simulink model "SST_FINAL_SIMULINK"  (R2017b)
settings: Solver=ode14x  StartTime=0.0  StopTime=120/60  MaxStep=1e-4  RelTol=1e-3
values from neighbouring files (symbols this model uses):
  C_3P4L = (Potencia_nominal)/(2*pi*60*0.1*((Entrada)^2))    (= 0.00858724363662)    [SST_FINAL.m]
  C_HB = 50000/(0.6*60*pi*(11397^2))    (= 3.40358447746e-06)    [SST_FINAL.m]
  ca = 1/(L*a)    [SST_FINAL.m]
  CDAB1 = 50*(Pnom/3)/(Vmin_DAB1^2*Fsw_DAB)    [SST_FINAL.m]
  CDAB2 = 50*(Pnom/3)/(Vmin_DAB2^2*Fsw_DAB)    [SST_FINAL.m]
  E = Nm*Vout_HB    (= 11397)    [SST_FINAL.m]
  Fsw_DAB = 30e3    (= 30000)    [SST_FINAL.m]
  Fsw_HB = 15e3    (= 15000)    [SST_FINAL.m]
  Fsw_NPC = 5040    [SST_FINAL.m]
  Inom_HB = (50e3/(13200*sqrt(3)))*sqrt(2)    [SST_FINAL.m]
  Kc_I = H_infI    [SST_FINAL.m]
  Kc_V = H_infV    [SST_FINAL.m]
  KcI_DAB = H_infI_DAB    [SST_FINAL.m]
  KcV_DAB = H_infV_DAB    [SST_FINAL.m]
  Ki = 2.5641    [SST_FINAL.m]
  Kp = 0.00138    [SST_FINAL.m]
  L = ((0.03*Entrada))/((2*pi*60)*(Imax))    [SST_FINAL.m]
  L_DAB = (1/Ntr)*VDAB1*VDAB2*D*(1-D)/(2*Fsw_DAB*(Pnom/3))    (= 2.89591875e-05)    [SST_FINAL.m]
  L_HB = 50e-3    (= 0.05)    [SST_FINAL.m]
  m = (2*Voltaje_pico)/Entrada    [SST_FINAL.m]
  Pnom = 50e3    (= 50000)    [SST_FINAL.m]
  R_DAB = 30e3*2*pi*L_DAB*0.1    (= 0.545867824224)    [SST_FINAL.m]
  R_HB = 120*pi*L_HB*0.05    (= 0.942477796077)    [SST_FINAL.m]
  R_LOAD2 = VDAB2^2/(Pnom/3)    (= 9.26694)    [SST_FINAL.m]
  tauI_I = 1/(2*pi*F_lagI)    (= 0.00265258238486)    [SST_FINAL.m]
  tauI_V = 1/(2*pi*F_LagV)    (= 0.00039788735773)    [SST_FINAL.m]
  tauII_DAB = 1/(2*pi*F_lagI_DAB)    (= 0.00265258238486)    [SST_FINAL.m]
  tauIV_DAB = 1/(2*pi*F_lagV_DAB)    (= 0.265258238486)    [SST_FINAL.m]
  Ts = 1/(200*Fsw_DAB)    (= 1.66666666667e-07)    [SST_FINAL.m]
  uLmt_dDAB = 0.5    [SST_FINAL.m]
  uLmt_I = 0.05    [SST_FINAL.m]
  uLmt_V = Inom_HB    [SST_FINAL.m]
  VDAB1 = 11397    [SST_FINAL.m]
  VDAB2 = 393    [SST_FINAL.m]
  Vp = Entrada/2    (= 196.5)    [SST_FINAL.m]
  W = 120*pi    (= 376.991118431)    [SST_FINAL.m]
  w = 120*pi    (= 376.991118431)    [SST_FINAL.m]
libraries: powerlib x102, powerlib_meascontrol x26, simulink x16, dspstat3 x3
(part 2 of 2)

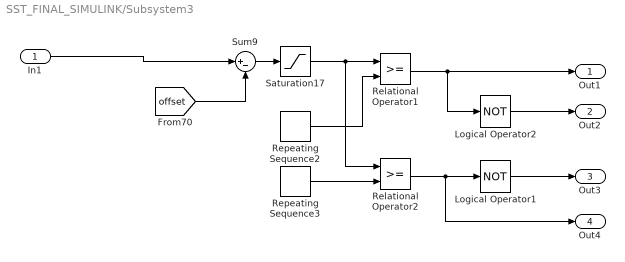
== system SST_FINAL_SIMULINK/Subsystem3 ==
  In1 : Inport
  Logical Operator1 : Logic  Operator=NOT  AllPortsSameDT=off  OutDataTypeStr=boolean
  Logical Operator2 : Logic  Operator=NOT  AllPortsSameDT=off  OutDataTypeStr=boolean
  Relational Operator1 : RelationalOperator  ZeroCross=off  RndMeth=Nearest
  Relational Operator2 : RelationalOperator  ZeroCross=off  RndMeth=Nearest
  Repeating Sequence2 : simulink/Sources/Repeating Sequence  rep_seq_t=[0 0.5/Fsw_NPC 1/Fsw_NPC]  rep_seq_y=[ 0 1 0 ]
  Repeating Sequence3 : simulink/Sources/Repeating Sequence  rep_seq_t=[0 0.5/Fsw_NPC 1/Fsw_NPC]  rep_seq_y=[-1 0 -1]
  Saturation17 : Saturate  UpperLimit=m  LowerLimit=-m  ZeroCross=off
  Sum9 : Sum  Inputs=|+-
  Out1 : Outport
  Out2 : Outport  Port=2
  Out3 : Outport  Port=3
  Out4 : Outport  Port=4
  wires:
  Saturation17/1 -> Relational Operator2/1, Relational Operator1/1
  Relational Operator1/1 -> Out1/1, Logical Operator2/1
  Repeating Sequence2/1 -> Relational Operator1/2
  Sum9/1 -> Saturation17/1
  Logical Operator2/1 -> Out2/1
  Logical Operator1/1 -> Out3/1
  [offset] -> Sum9/2
  Relational Operator2/1 -> Out4/1, Logical Operator1/1
  In1/1 -> Sum9/1
  Repeating Sequence3/1 -> Relational Operator2/2

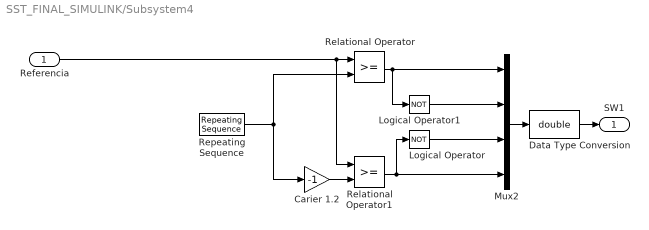
== system SST_FINAL_SIMULINK/Subsystem4 ==
  Referencia : Inport
  Carier 1.2 : Gain  Gain=-1
  Data Type Conversion : DataTypeConversion  OutDataTypeStr=double
  Logical Operator : Logic  Operator=NOT  IconShape=distinctive  AllPortsSameDT=off  OutDataTypeStr=boolean
  Logical Operator1 : Logic  Operator=NOT  IconShape=distinctive  AllPortsSameDT=off  OutDataTypeStr=boolean
  Mux2 : Mux
  Relational Operator : RelationalOperator  OutDataTypeStr=boolean  RndMeth=Simplest
  Relational Operator1 : RelationalOperator  OutDataTypeStr=boolean  RndMeth=Simplest
  Repeating Sequence : simulink/Sources/Repeating Sequence  rep_seq_t=[0 0.5 1]/Fsw_HB  rep_seq_y=[0 1 0]
  SW1 : Outport
  wires:
  Referencia/1 -> Relational Operator/1, Relational Operator1/1
  Repeating Sequence/1 -> Carier 1.2/1, Relational Operator/2
  Logical Operator1/1 -> Mux2/2
  Data Type Conversion/1 -> SW1/1
  Mux2/1 -> Data Type Conversion/1
  Logical Operator/1 -> Mux2/3
  Relational Operator/1 -> Mux2/1, Logical Operator1/1
  Carier 1.2/1 -> Relational Operator1/2
  Relational Operator1/1 -> Mux2/4, Logical Operator/1

== system SST_FINAL_SIMULINK/Subsystem5 ==
  In1 : Inport
  In2 : Inport  Port=2
  IGBT3 : powerlib/Power Electronics/IGBT  Ron=0.000000001  Lon=0  Vf=0  Tf=1e-6  Tt=2e-6  IC=0  Rs=inf  Cs=inf  Measurements=off
  IGBT4 : powerlib/Power Electronics/IGBT  Ron=0.000000001  Lon=0  Vf=0  Tf=1e-6  Tt=2e-6  IC=0  Rs=1e5  Cs=inf  Measurements=off
  Conn1 : PMIOPort  Port=1  Side=Left
  Conn2 : PMIOPort  Port=2  Side=Right
  Conn3 : PMIOPort  Port=3  Side=Left
  wires:
  In1/1 -> IGBT3/1
  In2/1 -> IGBT4/1
  connections:
  Conn3/RConn1 -- IGBT4/LConn1 -- IGBT3/RConn1
  IGBT4/RConn1 -- Conn2/RConn1
  IGBT3/LConn1 -- Conn1/RConn1

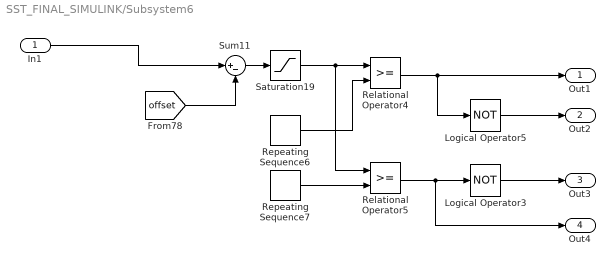
== system SST_FINAL_SIMULINK/Subsystem6 ==
  In1 : Inport
  Logical Operator3 : Logic  Operator=NOT  AllPortsSameDT=off  OutDataTypeStr=boolean
  Logical Operator5 : Logic  Operator=NOT  AllPortsSameDT=off  OutDataTypeStr=boolean
  Relational Operator4 : RelationalOperator  ZeroCross=off  RndMeth=Nearest
  Relational Operator5 : RelationalOperator  ZeroCross=off  RndMeth=Nearest
  Repeating Sequence6 : simulink/Sources/Repeating Sequence  rep_seq_t=[0 0.5/Fsw_NPC 1/Fsw_NPC]  rep_seq_y=[ 0 1 0 ]
  Repeating Sequence7 : simulink/Sources/Repeating Sequence  rep_seq_t=[0 0.5/Fsw_NPC 1/Fsw_NPC]  rep_seq_y=[-1 0 -1]
  Saturation19 : Saturate  UpperLimit=m  LowerLimit=-m  ZeroCross=off
  Sum11 : Sum  Inputs=|+-
  Out1 : Outport
  Out2 : Outport  Port=2
  Out3 : Outport  Port=3
  Out4 : Outport  Port=4
  wires:
  Sum11/1 -> Saturation19/1
  Relational Operator5/1 -> Out4/1, Logical Operator3/1
  Logical Operator3/1 -> Out3/1
  Saturation19/1 -> Relational Operator5/1, Relational Operator4/1
  In1/1 -> Sum11/1
  [offset] -> Sum11/2
  Repeating Sequence6/1 -> Relational Operator4/2
  Repeating Sequence7/1 -> Relational Operator5/2
  Relational Operator4/1 -> Out1/1, Logical Operator5/1
  Logical Operator5/1 -> Out2/1

== system SST_FINAL_SIMULINK/Subsystem7 ==
  In1 : Inport
  In2 : Inport  Port=2
  IGBT1 : powerlib/Power Electronics/IGBT  Ron=0.000000001  Lon=0  Vf=0  Tf=1e-6  Tt=2e-6  IC=0  Rs=1e5  Cs=inf  Measurements=off
  IGBT3 : powerlib/Power Electronics/IGBT  Ron=0.000000001  Lon=0  Vf=0  Tf=1e-6  Tt=2e-6  IC=0  Rs=inf  Cs=inf  Measurements=off
  Conn1 : PMIOPort  Port=1  Side=Left
  Conn2 : PMIOPort  Port=2  Side=Right
  Conn3 : PMIOPort  Port=3  Side=Left
  wires:
  In1/1 -> IGBT3/1
  In2/1 -> IGBT1/1
  connections:
  Conn3/RConn1 -- IGBT3/RConn1 -- IGBT1/LConn1
  IGBT1/RConn1 -- Conn2/RConn1
  IGBT3/LConn1 -- Conn1/RConn1

== system SST_FINAL_SIMULINK/Subsystem8 ==
  In1 : Inport
  In2 : Inport  Port=2
  IGBT3 : powerlib/Power Electronics/IGBT  Ron=0.000000001  Lon=0  Vf=0  Tf=1e-6  Tt=2e-6  IC=0  Rs=1e5  Cs=inf  Measurements=off
  IGBT4 : powerlib/Power Electronics/IGBT  Ron=0.000000001  Lon=0  Vf=0  Tf=1e-6  Tt=2e-6  IC=0  Rs=inf  Cs=inf  Measurements=off
  Conn1 : PMIOPort  Port=1  Side=Left
  Conn2 : PMIOPort  Port=2  Side=Right
  Conn3 : PMIOPort  Port=3  Side=Left
  wires:
  In2/1 -> IGBT3/1
  In1/1 -> IGBT4/1
  connections:
  IGBT4/LConn1 -- Conn1/RConn1
  IGBT3/RConn1 -- Conn2/RConn1
  Conn3/RConn1 -- IGBT3/LConn1 -- IGBT4/RConn1

== system SST_FINAL_SIMULINK/Subsystem9 ==
  In1 : Inport
  In2 : Inport  Port=2
  IGBT3 : powerlib/Power Electronics/IGBT  Ron=0.000000001  Lon=0  Vf=0  Tf=1e-6  Tt=2e-6  IC=0  Rs=inf  Cs=inf  Measurements=off
  IGBT4 : powerlib/Power Electronics/IGBT  Ron=0.000000001  Lon=0  Vf=0  Tf=1e-6  Tt=2e-6  IC=0  Rs=1e5  Cs=inf  Measurements=off
  Conn1 : PMIOPort  Port=1  Side=Left
  Conn2 : PMIOPort  Port=2  Side=Right
  Conn3 : PMIOPort  Port=3  Side=Left
  wires:
  In2/1 -> IGBT4/1
  In1/1 -> IGBT3/1
  connections:
  IGBT3/LConn1 -- Conn1/RConn1
  IGBT4/RConn1 -- Conn2/RConn1
  Conn3/RConn1 -- IGBT4/LConn1 -- IGBT3/RConn1

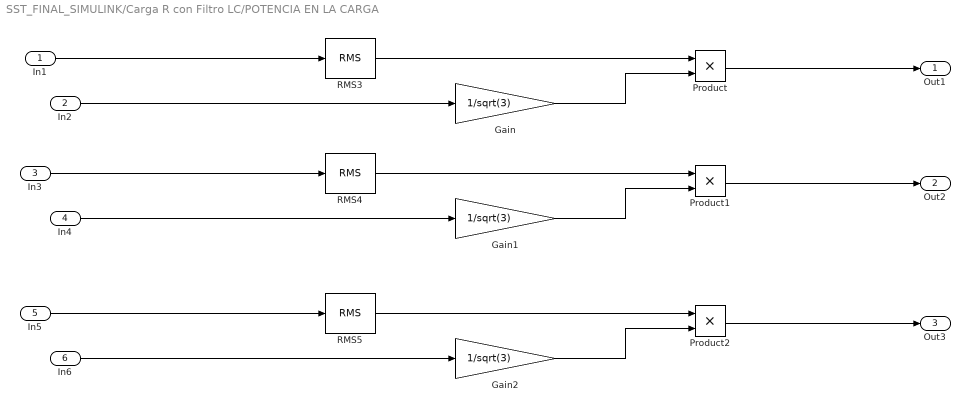
== system SST_FINAL_SIMULINK/Carga R con Filtro LC/POTENCIA EN LA CARGA  ==
  In1 : Inport
  In2 : Inport  Port=2
  In3 : Inport  Port=3
  In4 : Inport  Port=4
  In5 : Inport  Port=5
  In6 : Inport  Port=6
  Gain : Gain  Gain=1/sqrt(3)
  Gain1 : Gain  Gain=1/sqrt(3)
  Gain2 : Gain  Gain=1/sqrt(3)
  Product : Product
  Product1 : Product
  Product2 : Product
  RMS3 : powerlib_meascontrol/Measurements/RMS  TrueRMS=off  Freq=60  RMSInit=0  Ts=0
  RMS4 : powerlib_meascontrol/Measurements/RMS  TrueRMS=off  Freq=60  RMSInit=0  Ts=0
  RMS5 : powerlib_meascontrol/Measurements/RMS  TrueRMS=off  Freq=60  RMSInit=0  Ts=0
  Out1 : Outport
  Out2 : Outport  Port=2
  Out3 : Outport  Port=3
  wires:
  Gain1/1 -> Product1/2
  In4/1 -> Gain1/1
  In6/1 -> Gain2/1
  Product2/1 -> Out3/1
  Gain/1 -> Product/2
  RMS4/1 -> Product1/1
  RMS5/1 -> Product2/1
  Product/1 -> Out1/1
  RMS3/1 -> Product/1
  In3/1 -> RMS4/1
  In1/1 -> RMS3/1
  Product1/1 -> Out2/1
  Gain2/1 -> Product2/2
  In2/1 -> Gain/1
  In5/1 -> RMS5/1

== matlab function SST_FINAL_SIMULINK/CONTROL_ID_buck2 ==
  settings: updateMethod=DISCRETE  sampleTime=Ts
  data: yCur input; uCur output; rCur input; KcV_DAB parameter; tauIV_DAB parameter; Ts parameter
function uCur= PIV(yCur,rCur,KcV_DAB,tauIV_DAB,Ts)

persistent uPast yPast rPast
if isempty(uPast),uPast=0;end
if isempty(yPast),yPast=0;end
if isempty(rPast),rPast=0;end

% uCur=uPast+Kc_v*((rCur-yCur)-(rPast-yPast))+(Kc_v*Ts/tauI_v)*(rCur-yCur)+Kd_v*((rCur-yCur)-(rPast-yPast))/Ts;
uCur=uPast+KcV_DAB*((rCur-yCur)-(rPast-yPast))+(KcV_DAB*Ts/tauIV_DAB)*(rCur-yCur);

uPast=uCur;
yPast=yCur;
rPast=rCur;

== matlab function SST_FINAL_SIMULINK/MATLAB Function5 ==
  settings: updateMethod=DISCRETE  sampleTime=Ts
  data: yCur input; uCur output; rCur input; Kc_I parameter; tauI_I parameter; Ts parameter; uLmt_I parameter
function uCur= PIV(yCur,rCur,Kc_I,tauI_I,Ts,uLmt_I)

persistent uPast yPast rPast
if isempty(uPast),uPast=0;end
if isempty(yPast),yPast=0;end
if isempty(rPast),rPast=0;end

uCur=uPast+Kc_I*((rCur-yCur)-(rPast-yPast))+(Kc_I*Ts/tauI_I)*(rCur-yCur);

if (uCur>uLmt_I)
uCur=uLmt_I;
end
if (uCur<-uLmt_I)
uCur= -uLmt_I;
end

uPast=uCur;
yPast=yCur;
rPast=rCur;

== matlab function SST_FINAL_SIMULINK/CONTROL_ID_buck3 ==
  settings: updateMethod=DISCRETE  sampleTime=Ts
  data: yCur input; uCur output; rCur input; KcV_DAB parameter; tauIV_DAB parameter; Ts parameter
function uCur= PIV(yCur,rCur,KcV_DAB,tauIV_DAB,Ts)

persistent uPast yPast rPast
if isempty(uPast),uPast=0;end
if isempty(yPast),yPast=0;end
if isempty(rPast),rPast=0;end

% uCur=uPast+Kc_v*((rCur-yCur)-(rPast-yPast))+(Kc_v*Ts/tauI_v)*(rCur-yCur)+Kd_v*((rCur-yCur)-(rPast-yPast))/Ts;
uCur=uPast+KcV_DAB*((rCur-yCur)-(rPast-yPast))+(KcV_DAB*Ts/tauIV_DAB)*(rCur-yCur);

uPast=uCur;
yPast=yCur;
rPast=rCur;

== matlab function SST_FINAL_SIMULINK/CONTROL_ID_buck5 ==
  settings: updateMethod=DISCRETE  sampleTime=Ts
  data: yCur input; uCur output; rCur input; KcI_DAB parameter; tauII_DAB parameter; Ts parameter; uLmt_dDAB parameter
function uCur= PIV(yCur,rCur,KcI_DAB,tauII_DAB,Ts,uLmt_dDAB)

persistent uPast yPast rPast
if isempty(uPast),uPast=0;end
if isempty(yPast),yPast=0;end
if isempty(rPast),rPast=0;end

% uCur=uPast+Kc_v*((rCur-yCur)-(rPast-yPast))+(Kc_v*Ts/tauI_v)*(rCur-yCur)+Kd_v*((rCur-yCur)-(rPast-yPast))/Ts;
uCur=uPast+KcI_DAB*((rCur-yCur)-(rPast-yPast))+(KcI_DAB*Ts/tauII_DAB)*(rCur-yCur);

if (uCur>uLmt_dDAB)
uCur=uLmt_dDAB;
end
if (uCur<-uLmt_dDAB)
uCur= -uLmt_dDAB;
end

uPast=uCur;
yPast=yCur;
rPast=rCur;

== matlab function SST_FINAL_SIMULINK/MATLAB Function2 ==
  settings: updateMethod=DISCRETE  sampleTime=Ts
  data: Carrier_dab input; S_dab output; d_dab input
function S_dab = fcn(Carrier_dab,d_dab)


    
if Carrier_dab>=0 && Carrier_dab<pi
    if d_dab>Carrier_dab
        S_dab=[1 0 0 1 0 1 1 0];
    else
        S_dab=[1 0 0 1 1 0 0 1];
    end
else
    if (d_dab+pi)>Carrier_dab
        S_dab=[0 1 1 0 1 0 0 1];
    else
        S_dab=[0 1 1 0 0 1 1 0];
    end
end

end

== matlab function SST_FINAL_SIMULINK/MATLAB Function3 ==
  settings: updateMethod=DISCRETE  sampleTime=Ts
  data: Carrier_dab input; S_dab output; d_dab input
function S_dab = fcn(Carrier_dab,d_dab)


    
if Carrier_dab>=0 && Carrier_dab<pi
    if d_dab>Carrier_dab
        S_dab=[1 0 0 1 0 1 1 0];
    else
        S_dab=[1 0 0 1 1 0 0 1];
    end
else
    if (d_dab+pi)>Carrier_dab
        S_dab=[0 1 1 0 1 0 0 1];
    else
        S_dab=[0 1 1 0 0 1 1 0];
    end
end

end

== matlab function SST_FINAL_SIMULINK/MATLAB Function6 ==
  settings: updateMethod=DISCRETE  sampleTime=Ts
  data: yCur input; uCur output; rCur input; Kc_I parameter; tauI_I parameter; Ts parameter; uLmt_I parameter
function uCur= PIV(yCur,rCur,Kc_I,tauI_I,Ts,uLmt_I)

persistent uPast yPast rPast
if isempty(uPast),uPast=0;end
if isempty(yPast),yPast=0;end
if isempty(rPast),rPast=0;end

uCur=uPast+Kc_I*((rCur-yCur)-(rPast-yPast))+(Kc_I*Ts/tauI_I)*(rCur-yCur);

if (uCur>uLmt_I)
uCur=uLmt_I;
end
if (uCur<-uLmt_I)
uCur= -uLmt_I;
end

uPast=uCur;
yPast=yCur;
rPast=rCur;

== matlab function SST_FINAL_SIMULINK/CONTROL_ID_buck6 ==
  settings: updateMethod=DISCRETE  sampleTime=Ts
  data: yCur input; uCur output; rCur input; KcI_DAB parameter; tauII_DAB parameter; Ts parameter; uLmt_dDAB parameter
function uCur= PIV(yCur,rCur,KcI_DAB,tauII_DAB,Ts,uLmt_dDAB)

persistent uPast yPast rPast
if isempty(uPast),uPast=0;end
if isempty(yPast),yPast=0;end
if isempty(rPast),rPast=0;end

% uCur=uPast+Kc_v*((rCur-yCur)-(rPast-yPast))+(Kc_v*Ts/tauI_v)*(rCur-yCur)+Kd_v*((rCur-yCur)-(rPast-yPast))/Ts;
uCur=uPast+KcI_DAB*((rCur-yCur)-(rPast-yPast))+(KcI_DAB*Ts/tauII_DAB)*(rCur-yCur);

if (uCur>uLmt_dDAB)
uCur=uLmt_dDAB;
end
if (uCur<-uLmt_dDAB)
uCur= -uLmt_dDAB;
end

uPast=uCur;
yPast=yCur;
rPast=rCur;

== matlab function SST_FINAL_SIMULINK/MATLAB Function4 ==
  settings: updateMethod=DISCRETE  sampleTime=Ts
  data: Carrier_dab input; S_dab output; d_dab input
function S_dab = fcn(Carrier_dab,d_dab)


    
if Carrier_dab>=0 && Carrier_dab<pi
    if d_dab>Carrier_dab
        S_dab=[1 0 0 1 0 1 1 0];
    else
        S_dab=[1 0 0 1 1 0 0 1];
    end
else
    if (d_dab+pi)>Carrier_dab
        S_dab=[0 1 1 0 1 0 0 1];
    else
        S_dab=[0 1 1 0 0 1 1 0];
    end
end

end

== matlab function SST_FINAL_SIMULINK/MATLAB Function7 ==
  settings: updateMethod=DISCRETE  sampleTime=Ts
  data: yCur input; uCur output; rCur input; Kc_V parameter; tauI_V parameter; Ts parameter; uLmt_V parameter
function uCur= PIV(yCur,rCur,Kc_V,tauI_V,Ts,uLmt_V)

persistent uPast yPast rPast
if isempty(uPast),uPast=0;end
if isempty(yPast),yPast=0;end
if isempty(rPast),rPast=0;end

uCur=uPast+Kc_V*((rCur-yCur)-(rPast-yPast))+(Kc_V*Ts/tauI_V)*(rCur-yCur);

if (uCur>uLmt_V)
uCur=uLmt_V;
end
if (uCur<-uLmt_V)
uCur= -uLmt_V;
end

uPast=uCur;
yPast=yCur;
rPast=rCur;

== matlab function SST_FINAL_SIMULINK/CONTROL_ID_buck8 ==
  settings: updateMethod=DISCRETE  sampleTime=Ts
  data: yCur input; uCur output; rCur input; KcI_DAB parameter; tauII_DAB parameter; Ts parameter; uLmt_dDAB parameter
function uCur= PIV(yCur,rCur,KcI_DAB,tauII_DAB,Ts,uLmt_dDAB)

persistent uPast yPast rPast
if isempty(uPast),uPast=0;end
if isempty(yPast),yPast=0;end
if isempty(rPast),rPast=0;end

% uCur=uPast+Kc_v*((rCur-yCur)-(rPast-yPast))+(Kc_v*Ts/tauI_v)*(rCur-yCur)+Kd_v*((rCur-yCur)-(rPast-yPast))/Ts;
uCur=uPast+KcI_DAB*((rCur-yCur)-(rPast-yPast))+(KcI_DAB*Ts/tauII_DAB)*(rCur-yCur);

if (uCur>uLmt_dDAB)
uCur=uLmt_dDAB;
end
if (uCur<-uLmt_dDAB)
uCur= -uLmt_dDAB;
end

uPast=uCur;
yPast=yCur;
rPast=rCur;

== matlab function SST_FINAL_SIMULINK/CONTROL_ID_buck9 ==
  settings: updateMethod=DISCRETE  sampleTime=Ts
  data: yCur input; uCur output; rCur input; KcV_DAB parameter; tauIV_DAB parameter; Ts parameter
function uCur= PIV(yCur,rCur,KcV_DAB,tauIV_DAB,Ts)

persistent uPast yPast rPast
if isempty(uPast),uPast=0;end
if isempty(yPast),yPast=0;end
if isempty(rPast),rPast=0;end

% uCur=uPast+Kc_v*((rCur-yCur)-(rPast-yPast))+(Kc_v*Ts/tauI_v)*(rCur-yCur)+Kd_v*((rCur-yCur)-(rPast-yPast))/Ts;
uCur=uPast+KcV_DAB*((rCur-yCur)-(rPast-yPast))+(KcV_DAB*Ts/tauIV_DAB)*(rCur-yCur);

uPast=uCur;
yPast=yCur;
rPast=rCur;
